simulink model "msync_bo"  (R2026a)
settings: Solver=VariableStepAuto  StopTime=t_sim  MaxStep=1e-4  MinStep=1e-10  RelTol=1e-4  AbsTol=1e-6
values from neighbouring files (symbols this model uses):
  f_frot = 1e-3    (= 0.001)    [init_machine_synchrone.m]
  Gamma_c = 1.0    (= 1)    [init_machine_synchrone.m]
  Ir_ref = 4    [init_machine_synchrone.m]
  J = m*R^2/2    (= 0.246615023307)    [init_machine_synchrone.m]
  kr = ws_nom / t_rampe    (= 3.14159265359)    [init_machine_synchrone.m]
  M0 = (V_ent/(2*mu0))*Ks*Kr    (= 0.010232805843)    [init_machine_synchrone.m]
  param_elec = [Rs ; Ls ; Rr ; Lr ; M0]    [init_machine_synchrone.m]
  Rr = 2.0    (= 2)    [init_machine_synchrone.m]
  theta0 = -pi/4    (= -0.785398163397)    [init_machine_synchrone.m]
  Usm = 230    [init_machine_synchrone.m]
  w0 = 0    [init_machine_synchrone.m]
  ws_nom = 2*pi*5    (= 31.4159265359)    [init_machine_synchrone.m]
  x_elec_0 = [i1_0; i2_0; Ir_0]    [init_machine_synchrone.m]
libraries: simulink x1

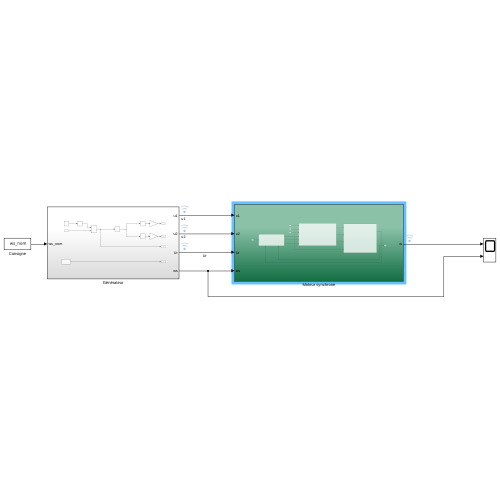
[thumbnail: Simulink's stored preview of the top-level diagram]
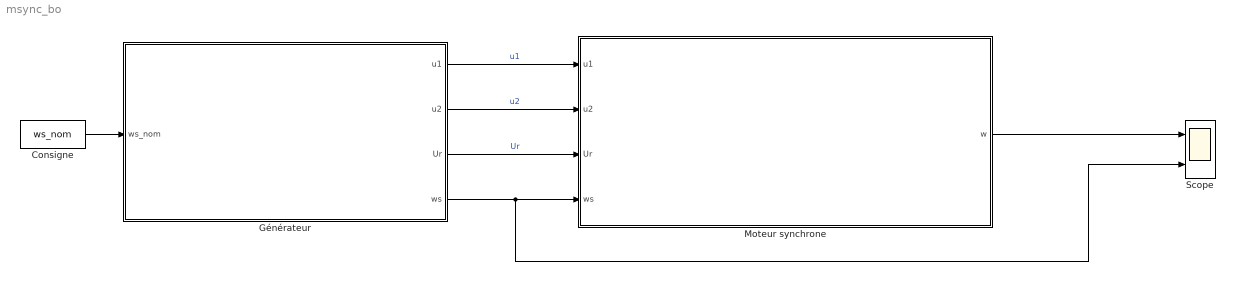
== system msync_bo ==
  Consigne : Constant  Value=ws_nom
  Générateur : Subsystem
  Moteur synchrone : Subsystem
  Scope : Scope  NumInputPorts=2
      settings: ActiveDisplayYMinimum=-8.9189480468527336  ActiveDisplayYMaximum=280.24367454652082
  wires:
  Générateur/4(ws) -> Moteur synchrone/4(ws), Scope/2
  Générateur/3(Ur) -> Moteur synchrone/3(Ur)  "Ur"
  Moteur synchrone/1(w) -> Scope/1
  Générateur/2(u2) -> Moteur synchrone/2(u2)  "u2"
  Générateur/1(u1) -> Moteur synchrone/1(u1)  "u1"
  Consigne/1 -> Générateur/1(ws_nom)

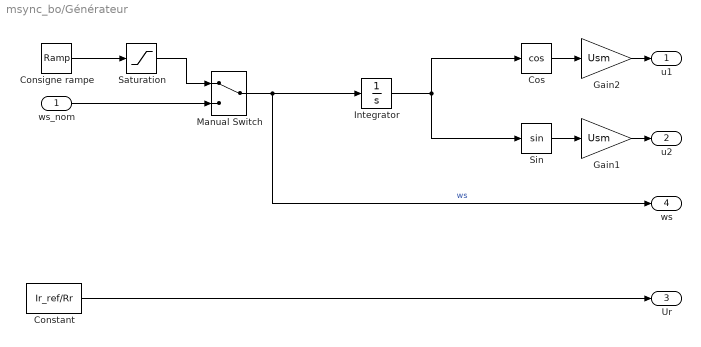
== system msync_bo/Générateur ==
  ws_nom : Inport
  Consigne rampe : simulink/Sources/Ramp  slope=kr  start=0  InitialOutput=20
  Constant : Constant  Value=Ir_ref/Rr
  Cos : Trigonometry  Operator=cos
  Gain1 : Gain  Gain=Usm
  Gain2 : Gain  Gain=Usm
  Integrator : Integrator
  Manual Switch : ManualSwitch
  Saturation : Saturate  UpperLimit=ws_nom  LowerLimit=-inf
  Sin : Trigonometry
  u1 : Outport
  u2 : Outport  Port=2
  Ur : Outport  Port=3
  ws : Outport  Port=4
  wires:
  Constant/1 -> Ur/1
  Cos/1 -> Gain2/1
  Sin/1 -> Gain1/1
  Integrator/1 -> Sin/1, Cos/1
  Gain2/1 -> u1/1
  Gain1/1 -> u2/1
  ws_nom/1 -> Manual Switch/2
  Consigne rampe/1 -> Saturation/1
  Manual Switch/1 -> ws/1, Integrator/1  "ws"
  Saturation/1 -> Manual Switch/1

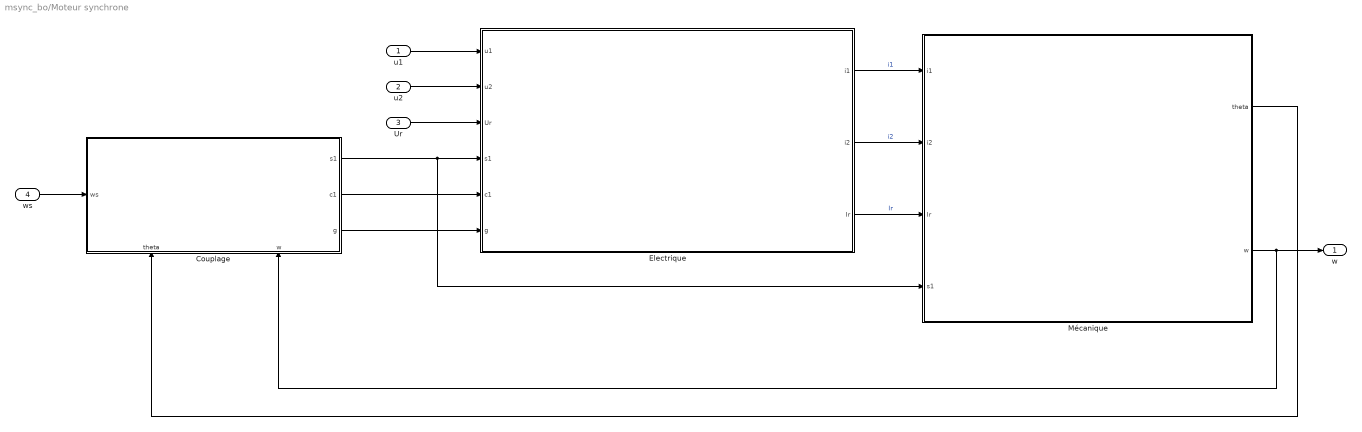
== system msync_bo/Moteur synchrone ==
  u1 : Inport
  u2 : Inport  Port=2
  Ur : Inport  Port=3
  ws : Inport  Port=4
  Couplage : Subsystem
      settings: PortSchema="{\"entries\":[{\"content\":{\"sides\":[{\"content\":{\"connectorIds\":[\"In1\"]},\"type\":\"ConnectorPlacement.EquallySpacedRectSide\",\"uuid\":\"9dc51e47-3ccd-4fcf-b58e-693782414d72\"},{\"content\":{\"connectorIds\":[\"Out1\",\"Out2\",\"Out3\"],\"side\":\"RIGHT\"},\"type\":\"ConnectorPlacement.EquallySpacedRectSide\",\"uuid\":\"19a88299-5411-4e53-b82f-2f137c46c168\"},{\"content\":{\"side\":\"TOP\"},\"type\":\"ConnectorPlacement.EquallySpacedRectSide\",\"uuid\":\"41370ab2-3a57-4936-8529-4b17c5065414\"},{\"content\":{\"connectorIds\":[\"In2\",\"In3\"],\"side\":\"BOTTOM\"},\"type\":\"ConnectorPlacement.EquallySpacedRectSide\",\"uuid\":\"3208a361-3d29-4bb8-a8eb-05b939f283cd\"}]},\"type\":\"ConnectorPlacement.EquallySpacedConnector\",\"uuid\":\"757f9aef-a381-4002-b608-7371e0c3c663\"}],\"packageUris\":[\"http://schema.mathworks.com/mf0/Connector/R2020b\"],\"version\":\"1.0\"}"
  Electrique : Subsystem
  Mécanique : Subsystem
  w : Outport
  wires:
  ws/1 -> Couplage/1(ws)
  Couplage/1(s1) -> Mécanique/4(s1), Electrique/4(s1)
  Couplage/3(g) -> Electrique/6(g)
  Mécanique/1(theta) -> Couplage/2(theta)
  Couplage/2(c1) -> Electrique/5(c1)
  Mécanique/2(w) -> w/1, Couplage/3(w)
  Ur/1 -> Electrique/3(Ur)
  u1/1 -> Electrique/1(u1)
  u2/1 -> Electrique/2(u2)
  Electrique/3(Ir) -> Mécanique/3(Ir)  "Ir"
  Electrique/1(i1) -> Mécanique/1(i1)  "i1"
  Electrique/2(i2) -> Mécanique/2(i2)  "i2"

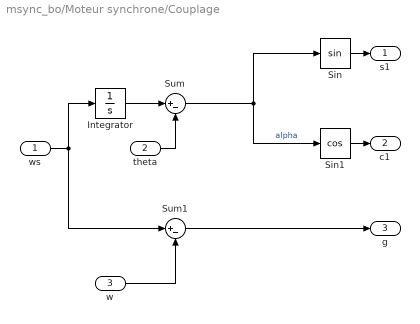
== system msync_bo/Moteur synchrone/Couplage ==
  ws : Inport
  theta : Inport  Port=2
  w : Inport  Port=3
  Integrator : Integrator
  Sin : Trigonometry
  Sin1 : Trigonometry  Operator=cos
  Sum : Sum  Inputs=|+-
  Sum1 : Sum  Inputs=|+-
  s1 : Outport
  c1 : Outport  Port=2
  g : Outport  Port=3
  wires:
  ws/1 -> Sum1/1, Integrator/1
  theta/1 -> Sum/2
  Integrator/1 -> Sum/1
  w/1 -> Sum1/2
  Sum/1 -> Sin1/1, Sin/1  "alpha"
  Sum1/1 -> g/1
  Sin/1 -> s1/1
  Sin1/1 -> c1/1

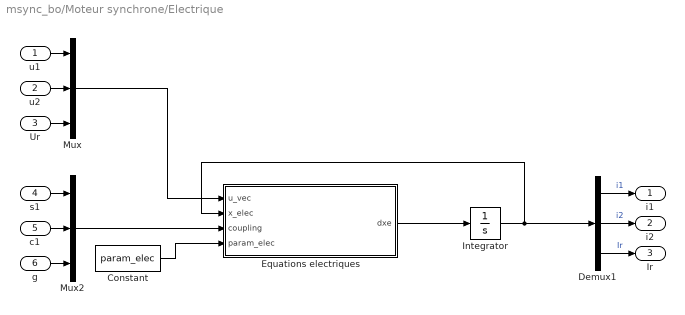
== system msync_bo/Moteur synchrone/Electrique ==
  u1 : Inport
  u2 : Inport  Port=2
  Ur : Inport  Port=3
  s1 : Inport  Port=4
  c1 : Inport  Port=5
  g : Inport  Port=6
  Constant : Constant  Value=param_elec
  Demux1 : Demux  Outputs=3
  Equations electriques : MATLAB Function  TreatAsAtomicUnit=on
  Integrator : Integrator  InitialCondition=x_elec_0
  Mux : Mux  Inputs=3
  Mux2 : Mux  Inputs=3
  i1 : Outport
  i2 : Outport  Port=2
  Ir : Outport  Port=3
  wires:
  s1/1 -> Mux2/1
  Equations electriques/1(dxe) -> Integrator/1
  Integrator/1 -> Demux1/1, Equations electriques/2(x_elec)
  Mux2/1 -> Equations electriques/3(coupling)
  c1/1 -> Mux2/2
  Mux/1 -> Equations electriques/1(u_vec)
  u1/1 -> Mux/1
  u2/1 -> Mux/2
  Ur/1 -> Mux/3
  g/1 -> Mux2/3
  Constant/1 -> Equations electriques/4(param_elec)
  Demux1/1 -> i1/1  "i1"
  Demux1/2 -> i2/1  "i2"
  Demux1/3 -> Ir/1  "Ir"

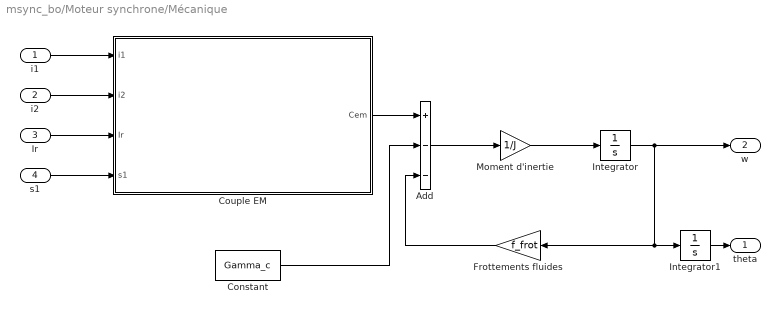
== system msync_bo/Moteur synchrone/Mécanique ==
  i1 : Inport
  i2 : Inport  Port=2
  Ir : Inport  Port=3
  s1 : Inport  Port=4
  Add : Sum  Inputs=+--
  Constant : Constant  Value=Gamma_c
  Couple EM : Subsystem
  Frottements fluides : Gain  Gain=f_frot
  Integrator : Integrator  InitialCondition=w0
  Integrator1 : Integrator  InitialCondition=theta0
  Moment d'inertie : Gain  Gain=1/J
  theta : Outport
  w : Outport  Port=2
  wires:
  Ir/1 -> Couple EM/3(Ir)
  Integrator/1 -> w/1, Integrator1/1, Frottements fluides/1
  i1/1 -> Couple EM/1(i1)
  Add/1 -> Moment d'inertie/1
  Moment d'inertie/1 -> Integrator/1
  Frottements fluides/1 -> Add/3
  s1/1 -> Couple EM/4(s1)
  Integrator1/1 -> theta/1
  i2/1 -> Couple EM/2(i2)
  Constant/1 -> Add/2
  Couple EM/1(Cem) -> Add/1

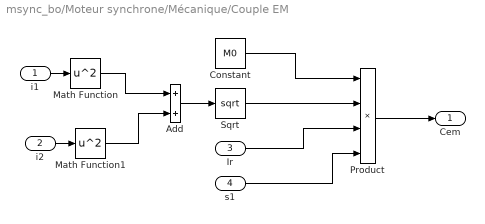
== system msync_bo/Moteur synchrone/Mécanique/Couple EM ==
  i1 : Inport
  i2 : Inport  Port=2
  Ir : Inport  Port=3
  s1 : Inport  Port=4
  Add : Sum
  Constant : Constant  Value=M0
  Math Function : Math  Operator=square
  Math Function1 : Math  Operator=square
  Product : Product  Inputs=4
  Sqrt : Sqrt
  Cem : Outport
  wires:
  Math Function/1 -> Add/1
  Math Function1/1 -> Add/2
  Add/1 -> Sqrt/1
  i2/1 -> Math Function1/1
  i1/1 -> Math Function/1
  Product/1 -> Cem/1
  Sqrt/1 -> Product/2
  Constant/1 -> Product/1
  Ir/1 -> Product/3
  s1/1 -> Product/4

== matlab function msync_bo/Moteur synchrone/Electrique/Equations electriques ==
  data: u_vec input; dxe output; x_elec input; coupling input; param_elec input
function dxe = electrical_equations(u_vec, x_elec, coupling, param_elec)

% Importation des paramètres depuis la workspace
Rs = param_elec(1);
Ls = param_elec(2);
Rr = param_elec(3);
Lr = param_elec(4);
M0 = param_elec(5);

% Extraction des signaux
u1 = u_vec(1); u2 = u_vec(2); Ur = u_vec(3);
i1 = x_elec(1); i2 = x_elec(2); Ir = x_elec(3);
s1 = coupling(1); % sin(ws*t-theta)
c1 = coupling(2); % cos(ws*t-theta)
g  = coupling(3); % ws*t - omega

Ism = sqrt(i1^2+i2^2);

% Phase statorique 1
di1 = (u1-Rs*i1-M0*Ir*g*s1)/Ls;

% Phase statorique 2
% Note: +cos car sin(ws*t-theta+pi/2) = cos(ws*t-theta)
di2 = (u2-Rs*i2+M0*Ir*g*c1)/Ls;

% Circuit rotorique
dIr = (Ur-Rr*Ir-M0*Ism*g*(-s1))/Lr;

% Vecteur de sortie
dxe = [di1 ; di2 ; dIr];
end
